simulink model "hexacopter"  (R2023b)
settings: Solver=ode3  StartTime=0.0  StopTime=inf  FixedStep=0.005  RelTol=1e-3
values from neighbouring files (symbols this model uses):
  A = [zeros(4),eye(4) ... (first row only)    [hexacopter_params.m]
  B = [0 0 0 0 ... (first row only)    [hexa.m]    (also in hexacopter_params.m = [zeros(4))
  body_params = [L,b,d,m,Ix,Iy,Iz,J_T]    [hexacopter_params.m]
  C = eye(8)    [hexacopter_params.m]
  g = 9.82    [hexacopter_params.m]
  K = place(A', C', desired_poles)'    [hexacopter_params.m]
  m = 2.5    [hexacopter_params.m]
  Simulation_params = [g,K_phi,K_theta,K_psi,K_x,K_y,K_z]    [hexacopter_params.m]
  T = [1, 1, 1, 1, 1, 1 ... (first row only)    [hexacopter_params.m]
  T_inv = pinv(T)    [hexacopter_params.m]
libraries: slpidlib x5, aerolibutil x2, vrlib x2
(part 2 of 2)

== matlab function hexacopter/Sliding mode controllers/MATLAB Function1 ==
  settings: updateMethod=DISCRETE
  data: x1 input; u output; x2 input; x1_d input; u_prev input
function u = SMC_Attitude(x1, x2, x1_d, u_prev)
% SMC with constant reference (assumes dx1_d = 0, ddx1_d = 0)

Iy = 100*0.00915; % moment of inertia x [kg*m^2]
h = 1/Iy;

f = 0;
% k      = 8;
% Gamma  = 18;
% delta  = 4;

k      = 1;
Gamma  = 20;
delta  = 0.1;

% k      = 0;
% Gamma  = 20*h;
% delta  = 0;

persistent z_i
if isempty(z_i)
    z_i = 0;
end
e = x1 - x1_d;
de = x2;  % dx1_d = 0
s = de + k * e;
d_hat = z_i + delta * x2;
dz = -delta * z_i - delta * (delta * x2 + f + h * u_prev);
z_i = z_i + dz * 0.005;  % 200 Hz
if abs(s) <= 1
    sat_s = s;
else
    sat_s = sign(s);
end
u = (-f - d_hat - k * de - Gamma * sat_s) / h;
